simulink model "SISOC_2016b"  (Simulink 8.8)
settings: Solver=ode45  StartTime=0.0  StopTime=tend  FixedStep=Tp  MaxStep=0.01  RelTol=1e-3  EnableMultiTasking=on
InitFcn:
  | Tp = 0.05;
  | sigma2e = 0.1;
  | TF = 8*Tp;
  | N = 20000;
  | tend = N*Tp;
  | Ro = 10;
  | global phat_RIV_n1 PIV_n1;
  | phat_RIV_n1 = zeros(3,1);
  | PIV_n1 = Ro*eye(3,3);
libraries: simulink x1
settings Model: Creator=kszygenda  LastModifiedBy=kszygenda
settings SolverCC: InsertRTBMode=Always
settings OptimizationCC: InitFltsAndDblsToZero=on
settings DebuggingCC: SaveWithParameterizedLinksMsg=none  SignalResolutionControl=TryResolveAllWithWarning  SolverPrmCheckMsg=warning  MultiTaskDSMMsg=warning  MultiTaskCondExecSysMsg=none  StateNameClashWarn=none
settings ModelReferenceCC: EnableRefExpFcnMdlSchedulingChecks=off
settings SFSimCC: SimUseLocalCustomCode=on
settings RTWCC: RTWUseLocalCustomCode=on
settings GRTTargetCC: TargetFcnLib=ansi_tfl_tmw.mat
settings ConfigComp: CovExternalEMLEnable=on

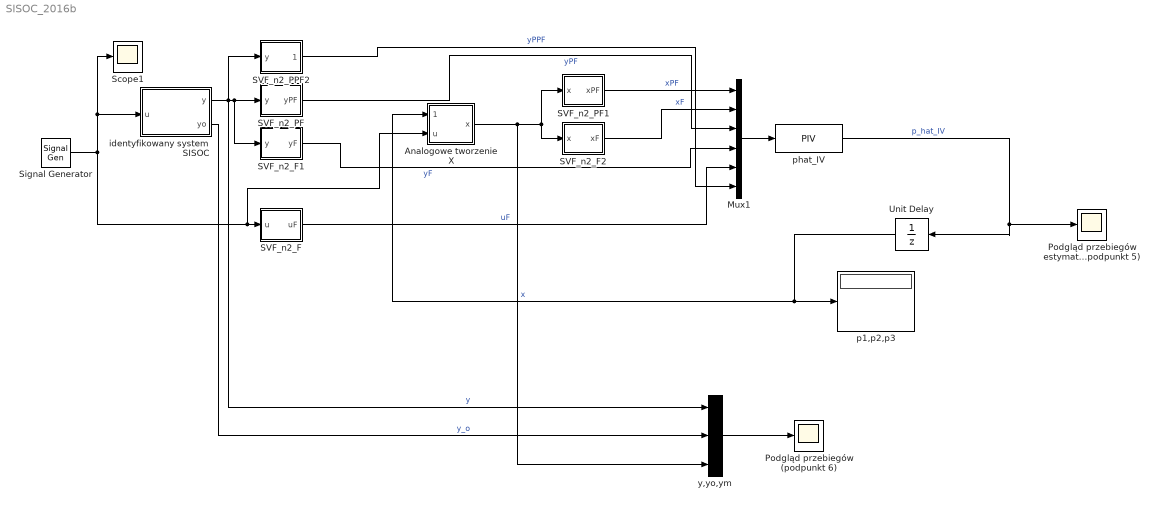
== system SISOC_2016b ==
  Analogowe tworzenie X : Subsystem
  Mux1 : Mux  Inputs=6
  Podgląd przebiegów (podpunkt 6) : Scope
  Podgląd przebiegów estymat (podpunkt 5) : Scope
  SVF_n2_F : Subsystem
  SVF_n2_F1 : Subsystem
  SVF_n2_F2 : Subsystem
  SVF_n2_PF : Subsystem
  SVF_n2_PF1 : Subsystem
  SVF_n2_PPF2 : Subsystem
  Scope1 : Scope
  Signal Generator : SignalGenerator  WaveForm=square  Frequency=0.04
  Unit Delay : UnitDelay  SampleTime=Tp  HasFrameUpgradeWarning=on
  identyfikowany system SISOC : Subsystem
  p1,p2,p3 : Display
  phat_IV : MATLABFcn  MATLABFcn=PIV  OutputDimensions=3  OutputSignalType=real
  y,yo,ym : Mux  Inputs=3
  wires:
  Signal Generator/1 -> SVF_n2_F/1(u), Analogowe tworzenie X/2(u), Scope1/1, identyfikowany system SISOC/1(u)
  identyfikowany system SISOC/1(y) -> SVF_n2_PPF2/1(y), SVF_n2_PF/1(y), SVF_n2_F1/1(y), y,yo,ym/1  "y"
  Analogowe tworzenie X/1(x) -> y,yo,ym/3, SVF_n2_F2/1(x), SVF_n2_PF1/1(x)  "x"
  Unit Delay/1 -> Analogowe tworzenie X/1(p_par), p1,p2,p3/1
  SVF_n2_F/1(uF) -> Mux1/5  "uF"
  SVF_n2_F1/1(yF) -> Mux1/4  "yF"
  SVF_n2_PF/1(yPF) -> Mux1/3  "yPF"
  SVF_n2_PF1/1(xPF) -> Mux1/1  "xPF"
  SVF_n2_F2/1(xF) -> Mux1/2  "xF"
  Mux1/1 -> phat_IV/1
  SVF_n2_PPF2/1(yPPF) -> Mux1/6  "yPPF"
  phat_IV/1 -> Podgląd przebiegów estymat (podpunkt 5)/1, Unit Delay/1  "p_hat_IV"
  y,yo,ym/1 -> Podgląd przebiegów (podpunkt 6)/1
  identyfikowany system SISOC/2(yo) -> y,yo,ym/2  "y_o"

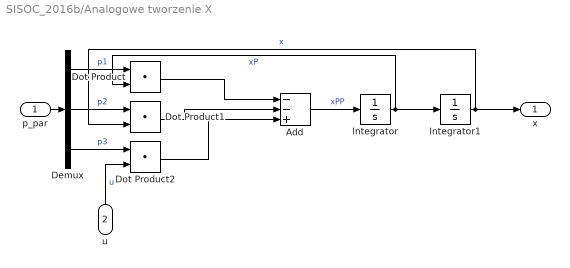
== system SISOC_2016b/Analogowe tworzenie X ==
  p_par : Inport
  u : Inport  Port=2
  Add : Sum  Inputs=--+
  Demux : Demux  Outputs=3
  Dot Product : DotProduct  InputSameDT=on  OutDataTypeStr=Inherit: Inherit via internal rule
  Dot Product1 : DotProduct  InputSameDT=on  OutDataTypeStr=Inherit: Inherit via internal rule
  Dot Product2 : DotProduct  InputSameDT=on  OutDataTypeStr=Inherit: Inherit via internal rule
  Integrator : Integrator
  Integrator1 : Integrator
  x : Outport
  wires:
  p_par/1 -> Demux/1
  Demux/3 -> Dot Product2/1  "p3"
  Dot Product2/1 -> Add/3
  Demux/2 -> Dot Product1/1  "p2"
  Demux/1 -> Dot Product/1  "p1"
  u/1 -> Dot Product2/2  "u"
  Dot Product1/1 -> Add/2
  Dot Product/1 -> Add/1
  Integrator/1 -> Dot Product/2, Integrator1/1  "xP"
  Integrator1/1 -> Dot Product1/2, x/1  "x"
  Add/1 -> Integrator/1  "xPP"

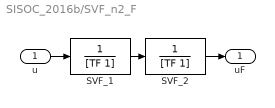
== system SISOC_2016b/SVF_n2_F ==
  u : Inport
  SVF_1 : TransferFcn  Denominator=[TF 1]
  SVF_2 : TransferFcn  Denominator=[TF 1]
  uF : Outport
  wires:
  SVF_1/1 -> SVF_2/1
  u/1 -> SVF_1/1
  SVF_2/1 -> uF/1

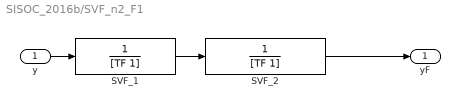
== system SISOC_2016b/SVF_n2_F1 ==
  y : Inport
  SVF_1 : TransferFcn  Denominator=[TF 1]
  SVF_2 : TransferFcn  Denominator=[TF 1]
  yF : Outport
  wires:
  SVF_1/1 -> SVF_2/1
  y/1 -> SVF_1/1
  SVF_2/1 -> yF/1

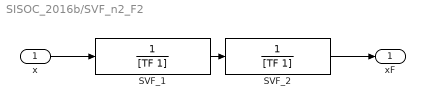
== system SISOC_2016b/SVF_n2_F2 ==
  x : Inport
  SVF_1 : TransferFcn  Denominator=[TF 1]
  SVF_2 : TransferFcn  Denominator=[TF 1]
  xF : Outport
  wires:
  SVF_1/1 -> SVF_2/1
  x/1 -> SVF_1/1
  SVF_2/1 -> xF/1

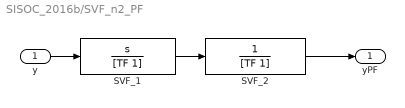
== system SISOC_2016b/SVF_n2_PF ==
  y : Inport
  SVF_1 : TransferFcn  Numerator=[1 0]  Denominator=[TF 1]
  SVF_2 : TransferFcn  Denominator=[TF 1]
  yPF : Outport
  wires:
  SVF_1/1 -> SVF_2/1
  y/1 -> SVF_1/1
  SVF_2/1 -> yPF/1

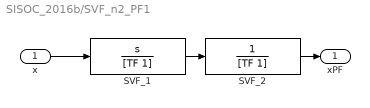
== system SISOC_2016b/SVF_n2_PF1 ==
  x : Inport
  SVF_1 : TransferFcn  Numerator=[1 0]  Denominator=[TF 1]
  SVF_2 : TransferFcn  Denominator=[TF 1]
  xPF : Outport
  wires:
  SVF_1/1 -> SVF_2/1
  x/1 -> SVF_1/1
  SVF_2/1 -> xPF/1

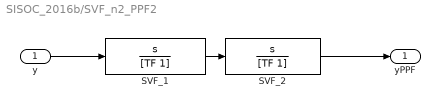
== system SISOC_2016b/SVF_n2_PPF2 ==
  y : Inport
  SVF_1 : TransferFcn  Numerator=[1 0]  Denominator=[TF 1]
  SVF_2 : TransferFcn  Numerator=[1 0]  Denominator=[TF 1]
  yPPF : Outport
  wires:
  SVF_1/1 -> SVF_2/1
  y/1 -> SVF_1/1
  SVF_2/1 -> yPPF/1

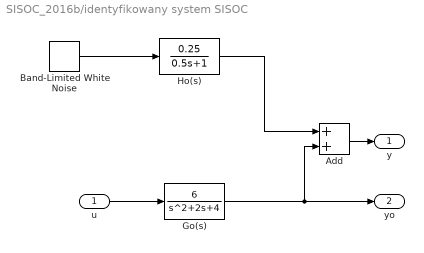
== system SISOC_2016b/identyfikowany system SISOC ==
  u : Inport
  Add : Sum
  Band-Limited White Noise : simulink/Sources/Band-Limited White Noise  Cov=[sigma2e]  Ts=Tp*0.1  seed=[2941]
  Go(s) : TransferFcn  Numerator=[6]  Denominator=[1 2 4]
  Ho(s) : TransferFcn  Numerator=[0.25]  Denominator=[0.5 1]
  y : Outport
  yo : Outport  Port=2
  wires:
  Band-Limited White Noise/1 -> Ho(s)/1
  Ho(s)/1 -> Add/1
  Go(s)/1 -> Add/2, yo/1
  Add/1 -> y/1
  u/1 -> Go(s)/1
